simulink model "Autonomous_Emergency_Braking"  (R2024a)
settings: Solver=VariableStepAuto  StartTime=0.0  StopTime=10.0  RelTol=1e-3
settings Model: DataDictionary=Autonomous_emergency_Breaking_data.sldd  Creator=kanna  LastModifiedBy=kanna
settings OptimizationCC: DefaultParameterBehavior=Inlined  EnhancedBackFolding=on  PassReuseOutputArgsAs=Individual arguments  ZeroExternalMemoryAtStartup=off  ZeroInternalMemoryAtStartup=off  OptimizeBlockOrder=speed  DifferentSizesBufferReuse=on  OptimizationCustomize=off  EfficientTunableParamExpr=on
settings DebuggingCC: ReadBeforeWriteMsg=DisableAll  WriteAfterWriteMsg=DisableAll  WriteAfterReadMsg=DisableAll  MultiTaskDSMMsg=none  ParameterTunabilityLossMsg=error
settings ModelReferenceCC: UpdateModelReferenceTargets=IfOutOfDate
settings SFSimCC: SFSimEcho=off  MATLABDynamicMemAlloc=off
settings RTWCC: Description=Embedded Coder  SystemTargetFile=ert.tlc  TemplateMakefile=ert_default_tmf  TargetLang=C++
settings CodeAppCC: ForceParamTrailComments=on  IgnoreCustomStorageClasses=off  OperatorAnnotations=on  SimulinkDataObjDesc=on  SFDataObjDesc=on  InsertBlockDesc=on
settings ERTTargetCC: TargetLangStandard=C++11 (ISO)  GenerateSampleERTMain=on  CodeInterfacePackaging=C++ class  InlinedParameterPlacement=NonHierarchical  RootIOFormat=Structure reference  ERTCustomFileTemplate=example_file_process.tlc

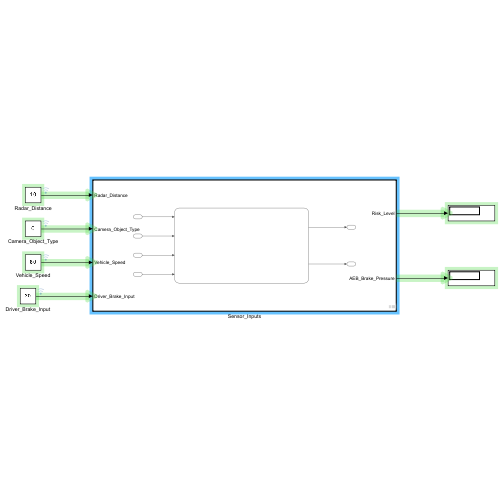
[thumbnail: Simulink's stored preview of the top-level diagram]
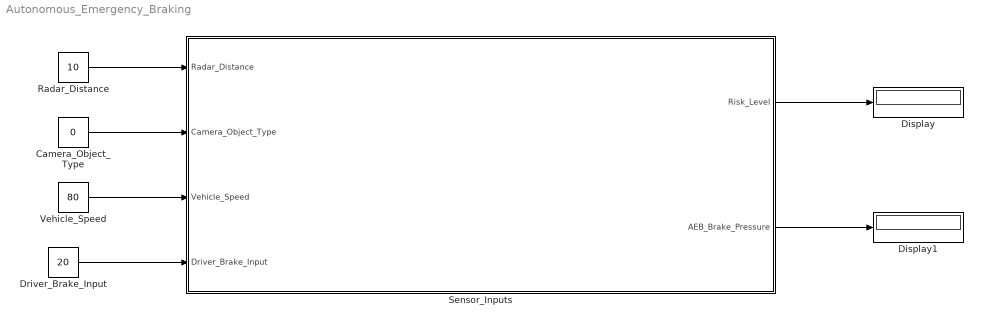
== system Autonomous_Emergency_Braking ==
  Camera_Object_Type : Constant  Value=0
  Display : Display
  Display1 : Display
  Driver_Brake_Input : Constant  Value=20
  Radar_Distance : Constant  Value=10
  Sensor_Inputs : Subsystem  TreatAsAtomicUnit=on
  Vehicle_Speed : Constant  Value=80
  wires:
  Radar_Distance/1 -> Sensor_Inputs/1(Radar_Distance)
  Camera_Object_Type/1 -> Sensor_Inputs/2(Camera_Object_Type)
  Vehicle_Speed/1 -> Sensor_Inputs/3(Vehicle_Speed)
  Driver_Brake_Input/1 -> Sensor_Inputs/4(Driver_Brake_Input)
  Sensor_Inputs/1(Risk_Level) -> Display/1
  Sensor_Inputs/2(AEB_Brake_Pressure) -> Display1/1

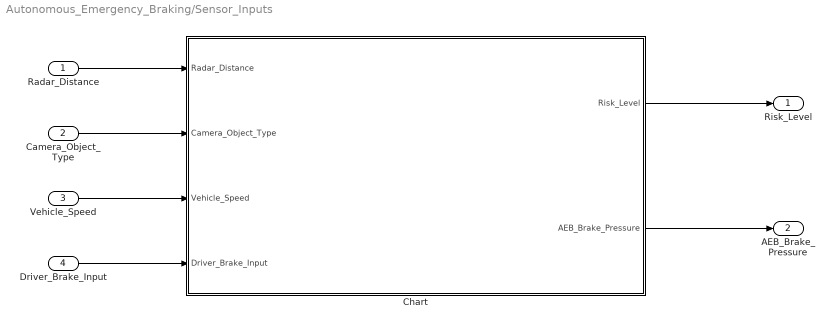
== system Autonomous_Emergency_Braking/Sensor_Inputs ==
  Radar_Distance : Inport
  Camera_Object_Type : Inport  Port=2
  Vehicle_Speed : Inport  Port=3
  Driver_Brake_Input : Inport  Port=4
  Chart : Stateflow chart  TreatAsAtomicUnit=on
  Risk_Level : Outport
  AEB_Brake_Pressure : Outport  Port=2
  wires:
  Radar_Distance/1 -> Chart/1(Radar_Distance)
  Camera_Object_Type/1 -> Chart/2(Camera_Object_Type)
  Vehicle_Speed/1 -> Chart/3(Vehicle_Speed)
  Chart/1(Risk_Level) -> Risk_Level/1
  Chart/2(AEB_Brake_Pressure) -> AEB_Brake_Pressure/1
  Driver_Brake_Input/1 -> Chart/4(Driver_Brake_Input)

== stateflow chart Autonomous_Emergency_Braking/Sensor_Inputs/Chart ==
  state Warning
    entry:
    Risk_Level=1;
    during :
    AEB_Brake_Pressure = Driver_Brake_Input;
  state Full_brake
    entry:
    Risk_Level=3;
    during :
    AEB_Brake_Pressure = 100;
  state Half_brake
    entry:
    Risk_Level=2;
    during :
    AEB_Brake_Pressure = 50;
  Warning -> Full_brake [order 3] : [[(Camera_Object_Type>0)&&...
      | ((Radar_Distance / (Vehicle_Speed + 0.1))<0.5)]]
  Full_brake -> Warning [order 3] : [[[(Camera_Object_Type>0)&&...
      | ((Radar_Distance / (Vehicle_Speed + 0.1))>1.5)]]]
  (default) -> Warning
  Full_brake -> Warning [order 1] : [[(Camera_Object_Type>0)&&...
      | ((Radar_Distance / (Vehicle_Speed + 0.1))>1.5)]]
  Warning -> Full_brake [order 1] : [[(Camera_Object_Type>0)&&...
      | ((Radar_Distance / (Vehicle_Speed + 0.1))<0.5)]]
  Full_brake -> Half_brake [order 2] : [(Camera_Object_Type>0)&&...
      | (((Radar_Distance / (Vehicle_Speed + 0.1))>0.5)&&...
      | ((Radar_Distance / (Vehicle_Speed + 0.1))<1.5))]
  Half_brake -> Full_brake [order 1] : [(Camera_Object_Type>0)&&...
      | ((Radar_Distance / (Vehicle_Speed + 0.1))<0.5)]
  Warning -> Half_brake [order 2] : [(Camera_Object_Type>0)&&...
      | (((Radar_Distance / (Vehicle_Speed + 0.1))>0.5)&&...
      | ((Radar_Distance / (Vehicle_Speed + 0.1))<1.5))]
  Half_brake -> Warning [order 2] : [[(Camera_Object_Type>0)&&...
      | ((Radar_Distance / (Vehicle_Speed + 0.1))>1.5)]]
  data: Radar_Distance input; Camera_Object_Type input; Vehicle_Speed input; Risk_Level output; AEB_Brake_Pressure output; Driver_Brake_Input input
